simulink library "DMS_slave_lib"  (Simulink 8.1)
settings: Solver=ode45  StartTime=0.0  StopTime=10.0  RelTol=1e-3
settings Model: Creator=ch24070  LastModifiedBy=pkoralew

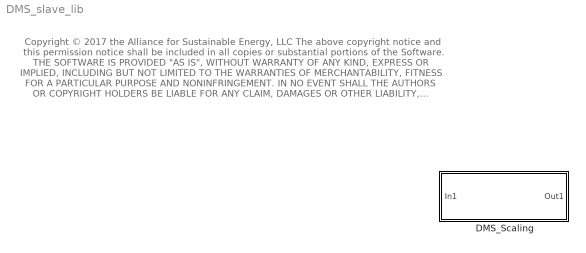
== system DMS_slave_lib ==
  note: Copyright © 2017 the Alliance for Sustainable Energy, LLC
      |
      | The above copyright notice and this permission notice shall be included in all copies or substantial portions of the Software.
      |
      | THE SOFTWARE IS PROVIDED "AS IS", WITHOUT WARRANTY OF ANY KIND, EXPRESS OR IMPLIED, INCLUDING
      | BUT NOT LIMITED TO THE WARRANTIES OF MERCHANTABILITY, FITNESS FOR A PARTICULAR PURPOSE AND
      | NONINFRINGEMENT. IN NO EVENT SHALL THE AUTHORS OR COPYRIGHT HOLDERS BE LIABLE FOR ANY CLAIM,
      |  DAMAGES OR OTHER LIABILITY, WHETHER IN AN ACTION OF CONTRACT, TORT OR OTHERWISE, ARISING FROM,
      | OUT OF OR IN CONNECTION WITH THE SOFTWARE OR THE USE OR OTHER DEALINGS IN THE SOFTWARE
  DMS_Scaling : Subsystem

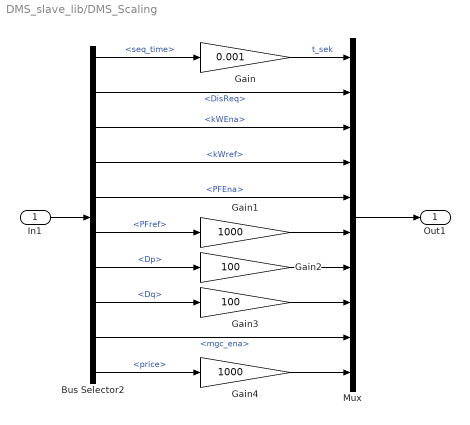
== system DMS_slave_lib/DMS_Scaling ==
  In1 : Inport
  Bus Selector2 : BusSelector  OutputSignals=seq_time,dms.DisReq,dms.kWEna,dms.kWref,dms.PFEna,dms.PFref,dms.Dp,dms.Dq,misc.mgc_ena,price
  Gain : Gain  Gain=0.001
  Gain1 : Gain  Gain=1000
  Gain2 : Gain  Gain=100
  Gain3 : Gain  Gain=100
  Gain4 : Gain  Gain=1000
  Mux : Mux  Inputs=10
  Out1 : Outport
  wires:
  Gain3/1 -> Mux/8
  Gain4/1 -> Mux/10
  Mux/1 -> Out1/1
  Bus Selector2/5 -> Mux/5  "<PFEna>"
  Bus Selector2/4 -> Mux/4  "<kWref>"
  Bus Selector2/6 -> Gain1/1  "<PFref>"
  Bus Selector2/10 -> Gain4/1  "<price>"
  Bus Selector2/8 -> Gain3/1  "<Dq>"
  Gain/1 -> Mux/1  "t_sek"
  Bus Selector2/3 -> Mux/3  "<kWEna>"
  Bus Selector2/9 -> Mux/9  "<mgc_ena>"
  Bus Selector2/7 -> Gain2/1  "<Dp>"
  Bus Selector2/2 -> Mux/2  "<DisReq>"
  Gain2/1 -> Mux/7
  Gain1/1 -> Mux/6
  Bus Selector2/1 -> Gain/1  "<seq_time>"
  In1/1 -> Bus Selector2/1
